simulink model "MySimplifiedTestingModel_2"  (R2023a)
settings: Solver=ode1  StartTime=0.0  StopTime=inf  FixedStep=0.001  RelTol=1e-3
PostLoadFcn:
  | , if any(exist('dsrtsu_mdlpostloadfcn', 'file') ~= 0), dsrtsu_mdlpostloadfcn('Execute', bdroot); end,
InitFcn:
  | , if any(exist('rtifpga_mdlclblib', 'file') ~= 0), rtifpga_mdlclblib('Init', bdroot); end,
model workspace (MAT data in the model file):
  mode = 2
libraries: rti1202serlib x5, simulink x2
(part 1 of 2)
Description:
  | Standard RTI1202 template.
  | Supported MATLAB version:  R2023a.
settings Model: Tag=RTI1202  DSRTSU_INTERNAL_RTI_VER=620  DSRTSU_INTERNAL_RTI_TYPE=rti1202  RTICANMMDATA=struct('GeneralSetupData',struct('modelroot','C:\Users\VM-User\Desktop\MigrationScripts','generalsettings',struct('filesettings',struct('destfolder',struct('Name','RTICANMM_FILES','Check',1),'buildfolder',struct('Name','.','Check',1),'AbsDestfolder',struct('Name','C:\Users\VM-User\Desktop\MigrationScripts\RTICANMM_FILES'),'AbsBuildfolder',struct('Name','C:\Users\VM-User\Desktop\MigrationScripts'))),'options',struct('addpaths',1,'rmpaths',1,'addtrcexclusion',true,'cannavigator',struct('checkmonitoring',0),'show_usrtrc',0,'use_usrtrc',0),'advanced',struct('options',ones(1,100)),'MPSetup',{{}},'RTI',struct('Type','RTI1202','Ver','7.17','Date','02-Nov-2021'),'modelname','','block','untitled'))  DSRTSU_INTERNAL_RTIFPGA=200  DSRTSU_INTERNAL_RTISTBM_VER=23.1  Creator=yd12yqyf  LastModifiedBy=ej62ixyv
settings SolverCC: AlgebraicLoopSolver=TrustRegion
settings DataIOCC: ReturnWorkspaceOutputs=off
settings OptimizationCC: BlockReduction=off  OptimizeBlockIOStorage=off  BufferReuse=off  ReuseModelBlockBuffer=off  GlobalBufferReuse=off  ExpressionFolding=off  LocalBlockOutputs=off  OptimizeDataStoreBuffers=off  BusAssignmentInplaceUpdate=off
settings DebuggingCC: UnderSpecifiedDataTypeMsg=warning  UnconnectedInputMsg=warning  UnconnectedOutputMsg=warning  UnconnectedLineMsg=warning  PregeneratedLibrarySubsystemCodeDiagnostic=none  UnderSpecifiedDimensionMsg=warning  ArithmeticOperatorsInVariantConditions=warning
settings HardwareCC: ProdBitPerPointer=32  ProdBitPerSizeT=32  ProdBitPerPtrDiffT=32  ProdLargestAtomicInteger=Integer  ProdEndianess=BigEndian  ProdWordSize=32  ProdLongLongMode=on  ProdHWDeviceType=Custom Processor->Custom  TargetIntDivRoundTo=Zero  TargetEndianess=BigEndian  TargetHWDeviceType=Custom Processor->Custom
settings ModelReferenceCC: EnableRefExpFcnMdlSchedulingChecks=on  EnableParallelModelReferenceBuilds=on  ParallelModelReferenceMATLABWorkerInit=Load Top Model
settings SFSimCC: SimUseLocalCustomCode=off  MATLABDynamicMemAlloc=off  CustomCodeUndefinedFunction=UseInterfaceOnly
settings RTWCC: Description=dSPACE DS1202 Hardware Platform  SystemTargetFile=rti1202.tlc  MakeCommand=make_rti  TemplateMakefile=rti1202.tmf  RTWUseLocalCustomCode=off  DLArmComputeVersion=19.05
settings CodeAppCC: StateflowObjectComments=on
settings STFCustomTargetCC: ParMdlRefBuildCompliant=on  ConcurrentExecutionCompliant=off  GRTInterface=off  UseToolchainInfoCompliant=off  SystemTargetFile=rti1202.tlc
settings GRTTargetCC: CompOptLevelCompliant=off  ConcurrentExecutionCompliant=off  CombineOutputUpdateFcns=off  MatFileLogging=off  CPPClassGenCompliant=off  UseToolchainInfoCompliant=off
settings ConfigComp: CovMetricSettings=dswe

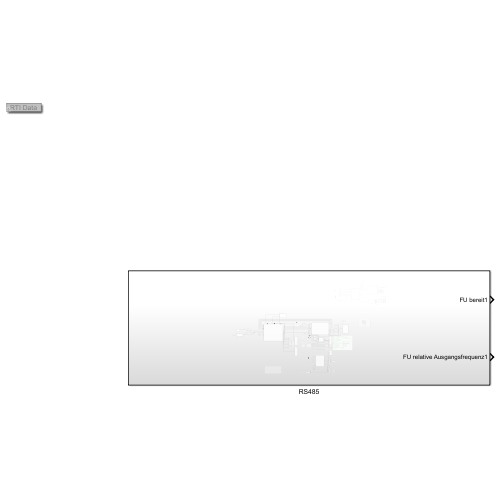
[thumbnail: Simulink's stored preview of the top-level diagram]
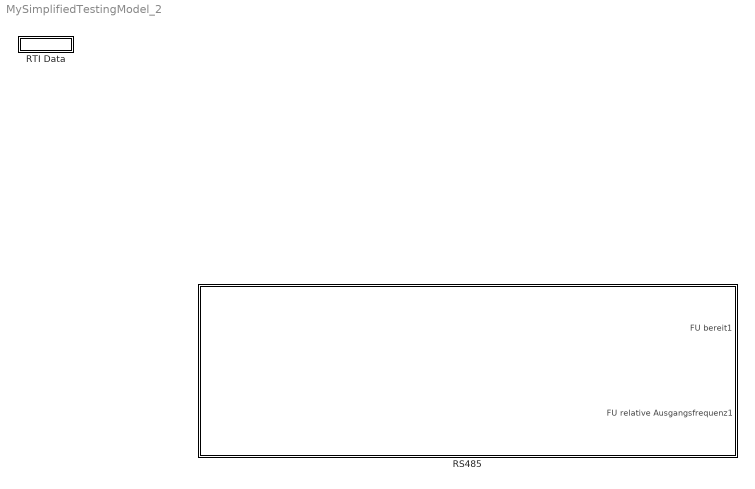
== system MySimplifiedTestingModel_2 ==
  RS485 : Subsystem
  RTI Data : Subsystem  Tag=struct('RTIDataServer',struct('RTIDataServerVs','2','RTIModelDescription','struct(''main'',''MySimplifiedTestingModel_2'',''sub'','''',''isMp'',0)'))  LoadFcn="if exist('rtidc'), try,  rtidc('DataHostBlockClbLoad', gcbh); catch, disp(['Warning: ''LoadFcn'' for RTI Data block failed: ' lasterr]); end, end,"  mask(RTI_DATA_HOST){}
      mask help:
      | RTI Data Block.
      | This block is used by RTI to store internal model-dependent data.
      | Please keep this block on the root level of the model. Deleting this block will result in data loss.
      |
      | NEVER DELETE OR COPY THIS BLOCK!
      settings: CopyFcn="if exist('rtidc'), try,  rtidc('DataHostBlockClbCopy', gcbh); catch, disp(['Warning: ''CopyFcn'' for RTI Data block failed: ' lasterr]); end, end,"  DeleteFcn="if exist('rtidc'), try,  rtidc('DataHostBlockClbDelete', gcbh); catch, disp(['Warning: ''DeleteFcn'' for RTI Data block failed: ' lasterr]); end, end,"  ModelCloseFcn="if exist('rtidc'), try,  rtidc('DataHostBlockClbModelClose', gcbh); catch, disp(['Warning: ''ModelCloseFcn'' for RTI Data block failed: ' lasterr]); end, end,"  PreSaveFcn="if exist('rtidc'), try,  rtidc('DataHostBlockClbPreSave', gcbh); catch, disp(['Warning: ''PreSaveFcn'' for RTI Data block failed: ' lasterr]); end, end,"  PostSaveFcn="if exist('rtidc'), try,  rtidc('DataHostBlockClbPostSave', gcbh); catch, disp(['Warning: ''PostSaveFcn'' for RTI Data block failed: ' lasterr]); end, end,"  NameChangeFcn="if exist('rtidc'), try,  rtidc('DataHostBlockClbNameChange', gcbh); catch, disp(['Warning: ''NameChangeFcn'' for RTI Data block failed: ' lasterr]); end, end,"
      mask Help:
      | RTI Data Block.
      | This block is used by RTI to store internal model-dependent data.
      | Please keep this block on the root level of the model. Deleting this block will result in data loss.
      | 
      | NEVER DELETE OR COPY THIS BLOCK!
      mask Display:
      | text(0.5, 0.5, 'RTI Data', 'HorizontalAlignment', 'center');
      | plot([1 0]);

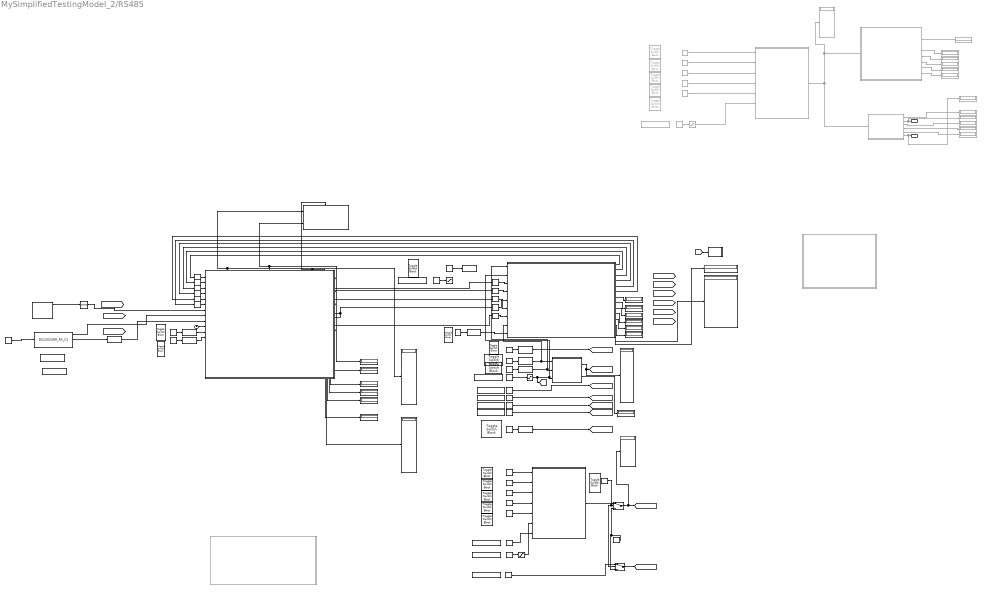
== system MySimplifiedTestingModel_2/RS485 ==
  note: RX_Data
  note: RX_Len
  note: THRE
  note: %| Bit| Bit value = 0 | Bit value = 1 |
      | %|----|--------------------------------------|------------------------------------|
      | %| 00 | selection between the four "3-10 Preset reference [0]...[3]" |
      | %| 01 | --""-- |
      | %|----|--------------------------------------|------------------------------------|
      | %| 02 | DC brake and stop | performs ramp |
      | %|----|--------------------------------------|------------------------------------|
      | %| 03 | lets the motor coast | starts the motor if conditions are met |
      | %|----|--------------------------------------|------------------------------------|
      | %| 04 | motor speed decreases until stop | |
      | %|----|--------------------------------------|------------------------------------|
      | %| 05 | current output frequency is stored | |
      | %|----|--------------------------------------|------------------------------------|
      | %| 06 | stop using ramp time | starts the motor if conditions are met |
      | %|----|--------------------------------------|------------------------------------|
      | %| 07 | no reset | reset |
      | %|----|--------------------------------------|------------------------------------|
      | %| 08 | | output frequency "3-19 Jog [RPM]" |
      | %|----|--------------------------------------|------------------------------------|
      | %| 09 | ramp 1 active ("3-41" and "3-42") | ramp 2 active ("3-51" and "3-52") |
      | %|----|--------------------------------------|------------------------------------|
      | %| 10 | control word is ignored | control word is used |
      | %|----|--------------------------------------|------------------------------------|
      | %| 11 | relay 01 not activated | relay 01 activated |
      | %|----|--------------------------------------|------------------------------------|
      | %| 12 | relay 04 not activated | relay 04 activated |
      | %|----|--------------------------------------|------------------------------------|
      | %| 13 | parameter set selection "0-10" and "8-55" |
      | %| 14 | |
      | %|----|--------------------------------------|------------------------------------|
      | %| 15 | no reversal | reversal |
  note: expect_len_ZKDM
  note: expect_crc_kind_ZKDM
  note: expect_addr_ZKDM
  note: req_len
  note: req_bytes
  note: req_valid
  note: resp_len
  note: resp_data
  note: resp_err_ZKDM
  note: resp_ok_ZKDM
  note: grant_ZKDM
  note: tx data
  note: tx len
  note: tx trigger
  Active : Constant  Value=0
  BUS MASTER FSM : Stateflow chart  TreatAsAtomicUnit=on
      settings: PortSchema="{\"entries\":[{\"content\":{\"sides\":[{\"content\":{\"connectorIds\":[\"In4\",\"In16\",\"In18\",\"In8\",\"In14\",\"In10\",\"In1\",\"In2\",\"In3\",\"In6\",\"In11\",\"In12\",\"In5\",\"In15\",\"In17\",\"In7\",\"In13\",\"In9\"]},\"type\":\"ConnectorPlacement.EquallySpacedRectSide\",\"uuid\":\"833d115e-8081-4cb1-98c4-083d374565ad\"},{\"content\":{\"connectorIds\":[\"Out4\",\"Out6\",\"Out5\",\"Out7\",\"Out9\",\"Out10\",\"Out11\",\"Out8\"],\"side\":\"RIGHT\"},\"type\":\"ConnectorPlacement.EquallySpacedRectSide\",\"uuid\":\"f0cbf871-5cea-4f22-8059-874c69130aa3\"},{\"content\":{\"connectorIds\":[\"Out1\",\"Out2\",\"Out3\"],\"side\":\"TOP\"},\"type\":\"ConnectorPlacement.EquallySpacedRectSide\",\"uuid\":\"9def79f2-ef8f-4b80-a903-98ac734b5ab3\"}]},\"type\":\"ConnectorPlacement.EquallySpacedConnector\",\"uuid\":\"db046b19-190e-410f-b654-5051c870f3be\"}],\"packageUris\":[\"http://schema.mathworks.com/mf0/Connector/R2020b\"],\"version\":\"1.0\"}"
  Begrenzung Arbeitstemperatur1 : Saturate  UpperLimit=100  LowerLimit=0  OutDataTypeStr=uint8
  Begrenzung Arbeitstemperatur2 : Saturate  Commented=on  UpperLimit=100  LowerLimit=0
  Begrenzung Arbeitstemperatur3 : Saturate  UpperLimit=100  LowerLimit=0
  Bit Index 6: Transmitter holding register empty (THRE) indicator1 : Selector  InputPortWidth=8  IndexOptions=Starting index (dialog)  Indices=[6]  OutputSizes=1
  Cast : DataTypeConversion  OutDataTypeStr=uint8  SaturateOnIntegerOverflow=off  RndMeth=Floor
  Cast To Boolean{,1..7} (8 alike) : DataTypeConversion  OutDataTypeStr=boolean  SaturateOnIntegerOverflow=off  RndMeth=Floor
  Clock : Clock
  Constant1 : Constant
  Constant10 : Constant
  Constant11 : Constant  Value=34
  Constant12 : Constant  Value=8  OutDataTypeStr=uint8
  Constant13 : Constant  Value=125
  Constant14 : Constant  Value=0
  Constant15 : Constant  Value=0  OutDataTypeStr=uint8
  Constant16 : Constant  Value=0
  Constant19 : Constant  Value=8  OutDataTypeStr=uint32
  Constant2 : Constant  Commented=on  Value=34
  Constant5 : Constant  Value=0
  Constant6 : Constant  Value=12  OutDataTypeStr=uint8
  Constant7 : Constant  Value=31  OutDataTypeStr=uint8
  Constant8 : Constant  Value=8  OutDataTypeStr=uint8
  ConstantSwitch{1,3..6} (5 alike) : Constant  Commented=on
  ConstantSwitch{2,8..11} (5 alike) : Constant  Value=0
  ConstantSwitch7 : Constant
  Create 8-Bytes Command : MATLAB Function  TreatAsAtomicUnit=on
  DS1202SER_RX_C2 : rti1202serlib/DS1202SER_RX_C1  Reserved1=[]  Reserved2=[]  Reserved3=[]  Reserved4=[]  DSProperties=struct('RTI',struct('IOBoardType',{{'DS1202','SER'}},'SlaveProcessor','NONE','Version',uint32(1),'BlockType',struct('isSLSource',uint8(1),'isSLSink',uint8(1),'isHWSource',uint8(0),'isHWSink',uint8(1),'isSetup',uint8(0),'isInline',uint8(1),'isNonInline',uint8(0),'isInterrupt',uint8(0),'isChannelwise',uint8(1)),'UnitType','GENSER','Identifier','RECEIVE','DialogType','ML','BlockSet','NONE'))  RTIBlockInterface=struct('BlockName',struct('Token',{{'DS1202SER_RX_C'}},'BlockParam',{{'ChannelNo'}}),'InputPortsWidth',int32(1),'InputPortsActive',1,'InputPortsDataType',{{'SS_UINT32'}},'InputPortsName',{{'NumBytes'}},'OutputPortsWidth',int32([127 1 1]),'OutputPortsActive',[1 1 1],'OutputPortsDataType',{{'SS_UINT8','SS_UINT32','SS_INT32'}},'OutputPortsName',{{'RXBytes','NumRXBytes','Status'}},'BlockDisplay',{{['Serial Receive'],'center'}},'IconTransparency','on','ParameterTunableNames',{{'BytesRefNumOf'}},'InitLevel',2,'DialogFcn','guigenserreceive','MaskDescription',['To read data from the UART SW FIFO.'])  RTIBlockParameters=struct('BoardNo',{{1,'ON',[1 1]}},'ChannelNo',{{2,'ON',[1 2]}},'ChannelNumOf',{{2,'OFF',[]}},'ReceptionDataMode',{{2,'OFF',[]}},'ParamTunableMode',{{1,'OFF',[]}},'BytesRefNumOfT',{{'1','OFF',[1 inf]}},'BytesRefNumOfNT',{{'1','OFF',[1 inf]}},'BytesRefNumOfMax',{{'127','OFF',[1 inf]}},'BytesRefNumOfMode',{{0,'OFF',[]}},'BytesActNumOfMode',{{1,'OFF',[]}},'ReceptionStatusMode',{{1,'OFF',[]}},'FifoSizeDefault',{{64,'OFF',[]}},'TLCFileName',{{'rtigenserreceive','OFF',[]}})  RTISFcnParameters=struct('BoardNo','double','ChannelNo','double','ChannelNumOf','double','ReceptionDataMode','double','ParamTunableMode','double','BytesRefNumOfT','double','BytesRefNumOfNT','double','BytesRefNumOfMax','double','BytesRefNumOfMode','double','BytesActNumOfMode','double','ReceptionStatusMode','double','TLCFileName','char')  RTIBlockParaDefault=struct('BoardNo',1,'ChannelNo',1,'ChannelNumOf',2,'ReceptionDataMode',1,'ParamTunableMode',1,'BytesRefNumOfT',1,'BytesRefNumOfNT',1,'BytesRefNumOfMax',1,'BytesRefNumOfMode',0,'BytesActNumOfMode',1,'ReceptionStatusMode',1,'FifoSizeDefault',64,'TLCFileName','rtigenserreceive')
  DS1202SER_SETUP_C1 : rti1202serlib/DS1202SER_SETUP_C1  Reserved1=[]  Reserved2=[]  Reserved3=[]  Reserved4=[]  DSProperties=struct('RTI',struct('Version',uint32(2),'IOBoardType',{{'DS1202','SER'}},'SlaveProcessor','NONE','BlockType',struct('isSLSource',uint8(0),'isSLSink',uint8(0),'isHWSource',uint8(0),'isHWSink',uint8(0),'isSetup',uint8(1),'isInline',uint8(1),'isNonInline',uint8(0),'isInterrupt',uint8(0),'isChannelwise',uint8(1)),'UnitType','GENSER','Identifier','SETUP','DialogType','ML','BlockSet','NONE'))  RTIBlockInterface=struct('BlockName',struct('Token',{{'DS1202SER_SETUP_C'}},'BlockParam',{{'ChannelNo'}}),'BlockDisplay',{{['Serial Setup'],'center'}},'IconTransparency','off','ParameterTunableNames',{{}},'InitLevel',1,'DialogFcn','guigensersetup','MaskDescription',['To set the global specifications for the UART interface.'])  RTIBlockParameters=struct('ParityMode',{{3,'OFF',[1 5]}},'TransceiverMode',{{[3;1],'OFF',[]}},'QuartzFrequency',{{'160000000','OFF',[]}},'BoardNo',{{1,'ON',[1 1]}},'ChannelNo',{{1,'ON',[1 2]}},'ChannelNumOf',{{2,'OFF',[]}},'BaudRate',{{'9600','OFF',[]}},'DataBitsNumOf',{{4,'OFF',[1 4]}},'StopBitsNumOf',{{1,'OFF',[1 3]}},'ReceiveIntLevelUart',{{1,'OFF',[1 4]}},'AutoflowMode',{{0,'OFF',[]}},'FifoSize',{{'128','OFF',[]}},'ReceiveIntLevelFifo',{{0,'OFF',[]}},'FifoOverrunMode',{{1,'OFF',[]}},'FifoBlockSize',{{'0','OFF',[]}},'TermMode',{{1,'OFF',[]}},'TLCFileName',{{'rtigensersetup','OFF',[]}})  RTISFcnParameters=struct('BoardNo','double','ChannelNo','double','ChannelNumOf','double','BaudRate','double','DataBitsNumOf','double','StopBitsNumOf','double','ParityMode','double','TransceiverMode','double','ReceiveIntLevelUart','double','AutoflowMode','double','FifoSize','double','ReceiveIntLevelFifo','double','FifoBlockSize','double','TermMode','double','QuartzFrequency','double','TLCFileName','char')  RTIBlockParaDefault=struct('ParityMode',1,'TransceiverMode',[1;1],'QuartzFrequency',160000000,'BoardNo',1,'ChannelNo',1,'ChannelNumOf',2,'BaudRate',115200,'DataBitsNumOf',4,'StopBitsNumOf',1,'ReceiveIntLevelUart',4,'AutoflowMode',0,'FifoSize',64,'ReceiveIntLevelFifo',0,'FifoOverrunMode',1,'FifoBlockSize',0,'TermMode',1,'TLCFileName','rtigensersetup')
  DS1202SER_SETUP_C2 : rti1202serlib/DS1202SER_SETUP_C1  Reserved1=[]  Reserved2=[]  Reserved3=[]  Reserved4=[]  DSProperties=struct('RTI',struct('Version',uint32(2),'IOBoardType',{{'DS1202','SER'}},'SlaveProcessor','NONE','BlockType',struct('isSLSource',uint8(0),'isSLSink',uint8(0),'isHWSource',uint8(0),'isHWSink',uint8(0),'isSetup',uint8(1),'isInline',uint8(1),'isNonInline',uint8(0),'isInterrupt',uint8(0),'isChannelwise',uint8(1)),'UnitType','GENSER','Identifier','SETUP','DialogType','ML','BlockSet','NONE'))  RTIBlockInterface=struct('BlockName',struct('Token',{{'DS1202SER_SETUP_C'}},'BlockParam',{{'ChannelNo'}}),'BlockDisplay',{{['Serial Setup'],'center'}},'IconTransparency','off','ParameterTunableNames',{{}},'InitLevel',1,'DialogFcn','guigensersetup','MaskDescription',['To set the global specifications for the UART interface.'])  RTIBlockParameters=struct('ParityMode',{{3,'OFF',[1 5]}},'TransceiverMode',{{[3;3],'OFF',[]}},'QuartzFrequency',{{'160000000','OFF',[]}},'BoardNo',{{1,'ON',[1 1]}},'ChannelNo',{{2,'ON',[1 2]}},'ChannelNumOf',{{2,'OFF',[]}},'BaudRate',{{'9600','OFF',[]}},'DataBitsNumOf',{{3,'OFF',[1 4]}},'StopBitsNumOf',{{1,'OFF',[1 3]}},'ReceiveIntLevelUart',{{1,'OFF',[1 4]}},'AutoflowMode',{{0,'OFF',[]}},'FifoSize',{{'128','OFF',[]}},'ReceiveIntLevelFifo',{{0,'OFF',[]}},'FifoOverrunMode',{{1,'OFF',[]}},'FifoBlockSize',{{'0','OFF',[]}},'TermMode',{{1,'OFF',[]}},'TLCFileName',{{'rtigensersetup','OFF',[]}})  RTISFcnParameters=struct('BoardNo','double','ChannelNo','double','ChannelNumOf','double','BaudRate','double','DataBitsNumOf','double','StopBitsNumOf','double','ParityMode','double','TransceiverMode','double','ReceiveIntLevelUart','double','AutoflowMode','double','FifoSize','double','ReceiveIntLevelFifo','double','FifoBlockSize','double','TermMode','double','QuartzFrequency','double','TLCFileName','char')  RTIBlockParaDefault=struct('ParityMode',1,'TransceiverMode',[1;1],'QuartzFrequency',160000000,'BoardNo',1,'ChannelNo',1,'ChannelNumOf',2,'BaudRate',115200,'DataBitsNumOf',4,'StopBitsNumOf',1,'ReceiveIntLevelUart',4,'AutoflowMode',0,'FifoSize',64,'ReceiveIntLevelFifo',0,'FifoOverrunMode',1,'FifoBlockSize',0,'TermMode',1,'TLCFileName','rtigensersetup')
  DS1202SER_STAT_C1 : rti1202serlib/DS1202SER_STAT_C1  Reserved1=[]  Reserved2=[]  Reserved3=[]  Reserved4=[]  DSProperties=struct('RTI',struct('IOBoardType',{{'DS1202','SER'}},'SlaveProcessor','NONE','Version',uint32(1),'BlockType',struct('isSLSource',uint8(1),'isSLSink',uint8(0),'isHWSource',uint8(0),'isHWSink',uint8(0),'isSetup',uint8(0),'isInline',uint8(1),'isNonInline',uint8(0),'isInterrupt',uint8(0),'isChannelwise',uint8(1)),'UnitType','GENSER','Identifier','STATUS','DialogType','ML','BlockSet','NONE'))  RTIBlockInterface=struct('BlockName',struct('Token',{{'DS1202SER_STAT_C'}},'BlockParam',{{'ChannelNo'}}),'OutputPortsWidth',int32([8 8 8]),'OutputPortsActive',[1 1 1],'OutputPortsName',{{'Line','Modem','Interrupt'}},'OutputPortsDataType',{{'SS_BOOLEAN','SS_BOOLEAN','SS_BOOLEAN'}},'BlockDisplay',{{['Serial Status'],'left'}},'IconTransparency','on','ParameterTunableNames',{{}},'InitLevel',1,'DialogFcn','guigenserstatus','MaskDescription',['To read the contents of the UART status register.'])  RTIBlockParameters=struct('BoardNo',{{1,'ON',[1 1]}},'ChannelNo',{{1,'ON',[1 2]}},'ChannelNumOf',{{2,'OFF',[]}},'LineStatUartMode',{{1,'OFF',[]}},'ModemStatUartMode',{{1,'OFF',[]}},'InterruptStatUartMode',{{1,'OFF',[]}},'TLCFileName',{{'rtigenserstatus','OFF',[]}})  RTISFcnParameters=struct('BoardNo','double','ChannelNo','double','ChannelNumOf','double','LineStatUartMode','double','ModemStatUartMode','double','InterruptStatUartMode','double','TLCFileName','char')  RTIBlockParaDefault=struct('BoardNo',1,'ChannelNo',1,'ChannelNumOf',2,'LineStatUartMode',1,'ModemStatUartMode',1,'InterruptStatUartMode',1,'TLCFileName','rtigenserstatus')
  Display{,1,9,16..31} (19 alike) : Display
      Display19 settings: Decimation=16
      Display21 settings: Decimation=16
      Display22 settings: Decimation=16
      Display25 settings: Decimation=8
      Display30 settings: Format=binary (Stored Integer)  Decimation=8
      Display31 settings: Format=binary (Stored Integer)
  Display{2..8,10..15} (13 alike) : Display  Commented=on
      Display15 settings: Decimation=8
  Edit{,3..10} (9 alike) : EditField  LabelPosition=Hide  ShowInitialText=on  Alignment=Center
  Edit2 : EditField  Commented=on  LabelPosition=Hide  ShowInitialText=on  Alignment=Center
  From : From
  Goto : Goto
  Invalid CTW : Constant  Value=0
  Length : Constant  Value=6  OutDataTypeStr=uint8
  MATLAB Function : MATLAB Function  TreatAsAtomicUnit=on
  MATLAB Function2 : MATLAB Function  Commented=on  TreatAsAtomicUnit=on
  MATLAB Function3 : MATLAB Function  Commented=on  TreatAsAtomicUnit=on
  MATLAB Function4 : MATLAB Function  TreatAsAtomicUnit=on
  Memory{,1..10} (11 alike) : Memory
  RX on : Constant  Value=0
  Saturation : Saturate  UpperLimit=100  LowerLimit=0
  Setpoint : Constant  Value=100
  Subsystem : Subsystem
  Subsystem2 : Subsystem  Commented=on
  Switch : Switch  Criteria=u2 > Threshold  SaturateOnIntegerOverflow=off  InputSameDT=off
  Switch1 : Switch  Criteria=u2 > Threshold  SaturateOnIntegerOverflow=off  InputSameDT=off
  THERMO FSM : Stateflow chart  Commented=on  TreatAsAtomicUnit=on
  TX on : Constant
  Toggle Switch{2,8..20} (14 alike) : ToggleSwitchBlock
      settings: Values={{'Off', 'On'}, [0 1]}
  Toggle Switch{3..7} (5 alike) : ToggleSwitchBlock  Commented=on
      settings: Values={{'Off', 'On'}, [0 1]}
  Variant Subsystem : Subsystem  Commented=on  Variant=on
  ZKDM FSM : Stateflow chart  TreatAsAtomicUnit=on
  FU bereit1 : Outport
  FU relative Ausgangsfrequenz1 : Outport  Port=2
  wires:
  Constant1/1 -> Begrenzung Arbeitstemperatur1/1
  Clock/1 -> BUS MASTER FSM/6(now)
  BUS MASTER FSM/4(grant_ZKDM) -> Memory/1, Display16/1
  BUS MASTER FSM/6(resp_ok_ZKDM) -> Memory1/1, Display17/1
  BUS MASTER FSM/5(resp_err_ZKDM) -> Memory2/1, Display18/1
  BUS MASTER FSM/7(resp_data) -> Display19/1, Memory3/1
  BUS MASTER FSM/9(resp_len) -> Memory4/1, Display20/1
  BUS MASTER FSM/1(TX_Data) -> Subsystem/1(TXBytes), Display22/1
  BUS MASTER FSM/2(TX_Len) -> Subsystem/2(NumBytes), Display23/1
  BUS MASTER FSM/3(TX_Trigger) -> Subsystem/Trigger, Display24/1
  ZKDM FSM/1(req_valid) -> Memory5/1
  ZKDM FSM/2(req_bytes) -> Memory6/1
  ZKDM FSM/3(req_len) -> Memory7/1
  ZKDM FSM/4(expect_addr_ZKDM) -> Memory8/1
  ZKDM FSM/6(expect_len_ZKDM) -> Memory9/1
  ZKDM FSM/5(expect_crc_kind_ZKDM) -> Memory10/1
  MATLAB Function3/1(u) -> Subsystem2/1(Antworttelegramm), Display15/1, MATLAB Function2/1(u)
  Begrenzung Arbeitstemperatur2/1 -> MATLAB Function3/6(freq_rel_percent)
  Constant2/1 -> Begrenzung Arbeitstemperatur2/1
  ConstantSwitch1/1 -> MATLAB Function3/1(fu_ctrl_ready)
  ConstantSwitch3/1 -> MATLAB Function3/2(fu_ready)
  ConstantSwitch4/1 -> MATLAB Function3/3(fault_trip)
  ConstantSwitch5/1 -> MATLAB Function3/4(fault_no_trip)
  ConstantSwitch6/1 -> MATLAB Function3/5(bus_control_active)
  MATLAB Function2/3(freq_rel_percent) -> Display2/1
  MATLAB Function2/5(fu_ctrl_ready) -> Display3/1
  MATLAB Function2/6(fu_ready) -> Display4/1
  MATLAB Function2/7(fault_trip) -> Display5/1
  MATLAB Function2/8(fault_no_trip) -> Display6/1
  MATLAB Function2/9(bus_control_active) -> Display7/1
  Subsystem2/5(Bussteuerung aktive) -> Display14/1
  Subsystem2/2(FU bereit) -> Display11/1, FU bereit1/1
  Subsystem2/1(Steuerung FU bereit) -> Display10/1
  Subsystem2/6(relative Ausgangsfrequenz) -> Display8/1, FU relative Ausgangsfrequenz1/1
  Subsystem2/3(Fehler mit Abschaltung) -> Display12/1
  Subsystem2/4(Fehler ohne Abschaltung) -> Display13/1
  Cast To Boolean/1 -> ZKDM FSM/8(invalid_flag), Create 8-Bytes Command/1(invalid_control_word)
  Cast To Boolean1/1 -> ZKDM FSM/1(active), Create 8-Bytes Command/2(active)
  Saturation/1 -> Goto/1, Create 8-Bytes Command/3(setpoint), ZKDM FSM/2(setpoint)
  Invalid CTW/1 -> Cast To Boolean/1
  Active/1 -> Cast To Boolean1/1
  Setpoint/1 -> Saturation/1
  Constant5/1 -> Cast To Boolean2/1
  Constant6/1 -> [expect_addr_ZKDM]
  Constant7/1 -> [expect_crc_kind_ZKDM]
  Constant8/1 -> [expect_len_ZKDM]
  Length/1 -> [req_len]
  Cast To Boolean2/1 -> [req_valid]
  Create 8-Bytes Command/1(command) -> Display21/1, [req_bytes]
  Cast To Boolean3/1 -> [THRE]
  Constant10/1 -> Cast To Boolean3/1
  Begrenzung Arbeitstemperatur3/1 -> MATLAB Function4/6(freq_rel_percent)
  ConstantSwitch10/1 -> MATLAB Function4/4(fault_no_trip)
  ConstantSwitch8/1 -> MATLAB Function4/2(fu_ready)
  ConstantSwitch11/1 -> MATLAB Function4/5(bus_control_active)
  Constant11/1 -> Begrenzung Arbeitstemperatur3/1
  ConstantSwitch7/1 -> MATLAB Function4/1(fu_ctrl_ready)
  MATLAB Function4/1(u) -> Switch/1
  ConstantSwitch9/1 -> MATLAB Function4/3(fault_trip)
  Constant12/1 -> Switch1/1
  Bit Index 6: Transmitter holding register empty (THRE) indicator1/1 -> BUS MASTER FSM/1(THRE)
  DS1202SER_RX_C2/1 -> BUS MASTER FSM/2(RX_Data)
  Constant13/1 -> MATLAB Function4/7(addr)
  Switch/1 -> Display25/1, [RX_Data]
  Constant14/1 -> Switch1/2, Switch/2
  Constant15/1 -> Switch1/3, Switch/3
  Switch1/1 -> [RX_Len]
  ConstantSwitch2/1 -> Cast To Boolean4/1
  Memory1/1 -> ZKDM FSM/4(resp_ok)
  Memory/1 -> ZKDM FSM/3(grant)
  Memory2/1 -> ZKDM FSM/6(resp_err)
  Memory3/1 -> ZKDM FSM/5(resp_data)
  Memory4/1 -> ZKDM FSM/7(resp_len)
  Memory5/1 -> BUS MASTER FSM/4(req_valid_ZKDM)
  Memory6/1 -> BUS MASTER FSM/16(req_bytes_ZKDM)
  Memory7/1 -> BUS MASTER FSM/18(req_len_ZKDM)
  Memory8/1 -> BUS MASTER FSM/8(expect_addr_ZKDM)
  Memory9/1 -> BUS MASTER FSM/14(expect_len_ZKDM)
  Memory10/1 -> BUS MASTER FSM/10(expect_crc_kind_ZKDM)
  Constant16/1 -> Cast To Boolean5/1
  Cast To Boolean5/1 -> ZKDM FSM/9(tx_trigger)
  Cast To Boolean6/1 -> BUS MASTER FSM/11(tx_switch)
  TX on/1 -> Cast To Boolean6/1
  Cast To Boolean7/1 -> BUS MASTER FSM/12(rx_switch)
  DS1202SER_STAT_C1/1 -> Bit Index 6: Transmitter holding register empty (THRE) indicator1/1
  Cast/1 -> BUS MASTER FSM/3(RX_Len)
  Constant19/1 -> DS1202SER_RX_C2/1
  DS1202SER_RX_C2/2 -> Cast/1
  ZKDM FSM/7(fault_no_trip) -> Display/1
  ZKDM FSM/8(fault_trip) -> Display1/1
  ZKDM FSM/9(fu_ctrl_ready) -> Display9/1
  ZKDM FSM/10(fu_ready) -> Display26/1
  ZKDM FSM/11(bus_ctrl_active) -> Display27/1
  ZKDM FSM/12(freq_rel) -> Display28/1
  RX on/1 -> Cast To Boolean7/1
  Create 8-Bytes Command/2(pcd2) -> Display29/1
  ZKDM FSM/13(debug_command) -> Display30/1
  From/1 -> MATLAB Function/1(setpoint)
  ZKDM FSM/14(debug_pcd2) -> Display31/1

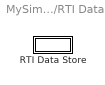
== system MySimplifiedTestingModel_2/RTI Data ==
  RTI Data Store : Subsystem  Tag="struct('private',struct('version',struct('dsVer',uint32(2)),'access',struct('modified',['19-Feb-2026 09:09:14'],'type','Model','isPerm',1)),'public',struct('main',struct('data',[]),'sub',struct('name',{{'MySimplifiedTestingModel_2'}},'data',{{struct('TH',struct('thTaskInfo',struct('taskType',{'TIMER','HWINT','TMRINT','SWINT','GLINT'},'tasksNumOf',{1,0,0,0,0},'srcIds',{{'TIMERA'},{},{},{},{}},'taskNames',{{['Timer Task 1']},{},{},{},{}})),'th_tc',struct('dataType','TASK','taskGroupId','','taskGroupList',{{}},'taskSchedulingPolicy','FCFS','taskType','TIMER','blkh',-1,'srcId','TIMERA','srcSgnName',['Timer A interrupt'],'srcCpuName','','taskName',['Timer Task 1  [0.001] s'],'taskNameDisplayExt','','smplTime',0.001,'smplTimeOffs',0,'hasFixedPriority',0,'priority',1,'hasFixedOvc',0,'ovcType',1,'ovcMax',1),'tc_th',struct('dataType','TASK','taskGroupId','','taskGroupList',{{}},'taskSchedulingPolicy','FCFS','taskType','TIMER','blkh',-1,'srcId','TIMERA','srcSgnName',['Timer A interrupt'],'srcCpuName','','taskName',['Timer Task 1  [0.001] s'],'taskNameDisplayExt','','smplTime',0.001,'smplTimeOffs',0,'hasFixedPriority',0,'priority',1,'hasFixedOvc',0,'ovcType',1,'ovcMax',1))}})))"  mask(RTI_DATA_STORE){}
      mask help:
      | RTI Data Store Block. This block is used by RTI to store internal model dependent data. Deleting this block will result in data loss.
      |
      | NEVER DELETE, COPY, OR MODIFY THIS BLOCK!
      mask Help:
      | RTI Data Store Block. This block is used by RTI to store internal model dependent data. Deleting this block will result in data loss.
      | 
      | NEVER DELETE, COPY, OR MODIFY THIS BLOCK!
      mask Display: text(0.5, 0.5, ' ', 'HorizontalAlignment', 'center');

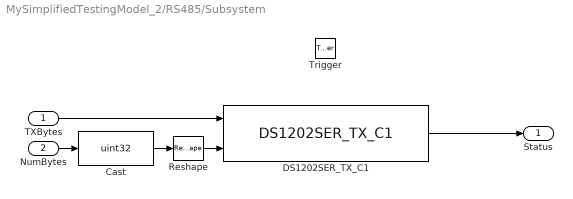
== system MySimplifiedTestingModel_2/RS485/Subsystem ==
  TXBytes : Inport
  NumBytes : Inport  Port=2
  Trigger : TriggerPort  VariantControl=(inherit)  PortDimensions=1
  Cast : DataTypeConversion  OutDataTypeStr=uint32  SaturateOnIntegerOverflow=off  RndMeth=Floor
  DS1202SER_TX_C1 : rti1202serlib/DS1202SER_TX_C1  Reserved1=[]  Reserved2=[]  Reserved3=[]  Reserved4=[]  DSProperties=struct('RTI',struct('IOBoardType',{{'DS1202','SER'}},'SlaveProcessor','NONE','Version',uint32(1),'BlockType',struct('isSLSource',uint8(1),'isSLSink',uint8(1),'isHWSource',uint8(1),'isHWSink',uint8(0),'isSetup',uint8(0),'isInline',uint8(1),'isNonInline',uint8(0),'isInterrupt',uint8(0),'isChannelwise',uint8(1)),'UnitType','GENSER','Identifier','TRANSMIT','DialogType','ML','BlockSet','NONE'))  RTIBlockInterface=struct('BlockName',struct('Token',{{'DS1202SER_TX_C'}},'BlockParam',{{'ChannelNo'}}),'InputPortsWidth',int32([127 1]),'InputPortsActive',[1 1],'InputPortsDataType',{{'SS_UINT8','SS_UINT32'}},'InputPortsName',{{'TXBytes','NumBytes'}},'OutputPortsWidth',int32([1 1]),'OutputPortsActive',[0 1],'OutputPortsDataType',{{'SS_UINT32','SS_INT32'}},'OutputPortsName',{{'NumTXBytes','Status'}},'BlockDisplay',{{['Serial Transmit'],'center'}},'IconTransparency','on','ParameterTunableNames',{{'BytesRefNumOf'}},'InitLevel',2,'DialogFcn','guigensertransmit','MaskDescription',['To write data to the UART SW FIFO.'])  RTIBlockParameters=struct('BoardNo',{{1,'ON',[1 1]}},'ChannelNo',{{1,'ON',[1 2]}},'ChannelNumOf',{{2,'OFF',[]}},'TransmitFifoOverrunMode',{{1,'OFF',[]}},'ParamTunableMode',{{1,'OFF',[]}},'BytesRefNumOfT',{{'32','OFF',[1 inf]}},'BytesRefNumOfNT',{{'64','OFF',[1 inf]}},'BytesRefNumOfMax',{{'127','OFF',[1 inf]}},'BytesRefNumOfMode',{{0,'OFF',[]}},'BytesActNumOfMode',{{0,'OFF',[]}},'TransmissionStatusMode',{{1,'OFF',[]}},'FifoSizeDefault',{{64,'OFF',[]}},'TLCFileName',{{'rtigensertransmit','OFF',[]}})  RTISFcnParameters=struct('BoardNo','double','ChannelNo','double','ChannelNumOf','double','TransmitFifoOverrunMode','double','ParamTunableMode','double','BytesRefNumOfT','double','BytesRefNumOfNT','double','BytesRefNumOfMax','double','BytesRefNumOfMode','double','BytesActNumOfMode','double','TransmissionStatusMode','double','TLCFileName','char')  RTIBlockParaDefault=struct('BoardNo',1,'ChannelNo',1,'ChannelNumOf',2,'TransmitFifoOverrunMode',1,'ParamTunableMode',1,'BytesRefNumOfT',1,'BytesRefNumOfNT',1,'BytesRefNumOfMax',1,'BytesRefNumOfMode',0,'BytesActNumOfMode',1,'TransmissionStatusMode',1,'FifoSizeDefault',64,'TLCFileName','rtigensertransmit')
  Reshape : Reshape
  Status : Outport
  wires:
  TXBytes/1 -> DS1202SER_TX_C1/1
  DS1202SER_TX_C1/1 -> Status/1
  NumBytes/1 -> Cast/1
  Cast/1 -> Reshape/1
  Reshape/1 -> DS1202SER_TX_C1/2

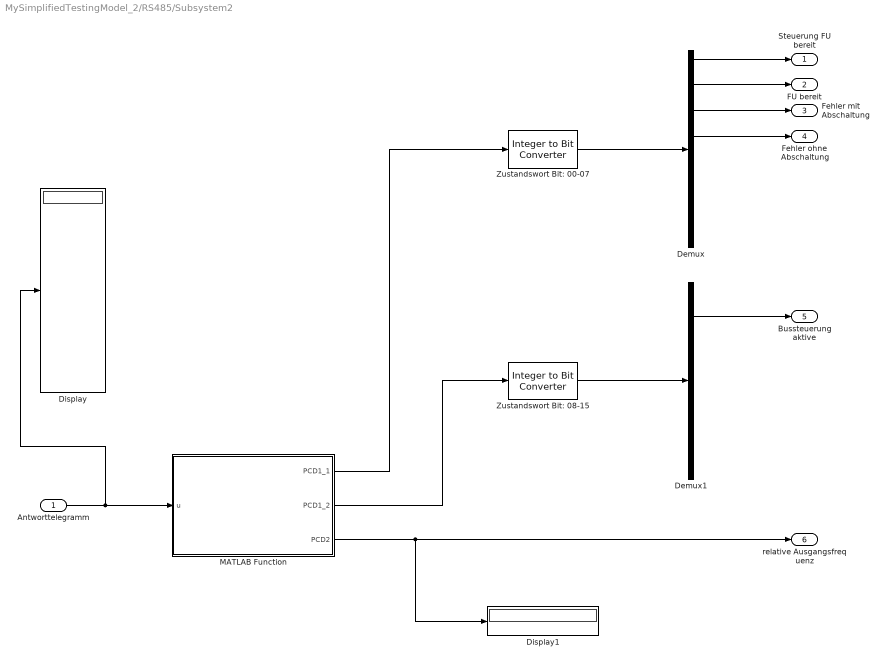
== system MySimplifiedTestingModel_2/RS485/Subsystem2 ==
  Antworttelegramm : Inport
  Demux : Demux  Outputs=8
  Demux1 : Demux  Outputs=8
  Display : Display
      settings: Decimation=8
  Display1 : Display
  MATLAB Function : MATLAB Function  TreatAsAtomicUnit=on
  Zustandswort Bit: 00-07 : simulink/Logic and Bit Operations/Integer to Bit Converter  nbits=8  signedInputValues=Unsigned  bitOrder=MSB first  outDtype=boolean
  Zustandswort Bit: 08-15 : simulink/Logic and Bit Operations/Integer to Bit Converter  nbits=8  signedInputValues=Unsigned  bitOrder=MSB first  outDtype=boolean
  Steuerung FU bereit : Outport
  FU bereit : Outport  Port=2
  Fehler mit Abschaltung : Outport  Port=3
  Fehler ohne Abschaltung : Outport  Port=4
  Bussteuerung aktive : Outport  Port=5
  relative Ausgangsfrequenz : Outport  Port=6
  wires:
  MATLAB Function/3(PCD2) -> Display1/1, relative Ausgangsfrequenz/1
  MATLAB Function/2(PCD1_2) -> Zustandswort Bit: 08-15/1
  MATLAB Function/1(PCD1_1) -> Zustandswort Bit: 00-07/1
  Demux1/2 -> Bussteuerung aktive/1
  Zustandswort Bit: 08-15/1 -> Demux1/1
  Zustandswort Bit: 00-07/1 -> Demux/1
  Demux/4 -> Fehler ohne Abschaltung/1
  Demux/3 -> Fehler mit Abschaltung/1
  Demux/2 -> FU bereit/1
  Demux/1 -> Steuerung FU bereit/1
  Antworttelegramm/1 -> Display/1, MATLAB Function/1(u)

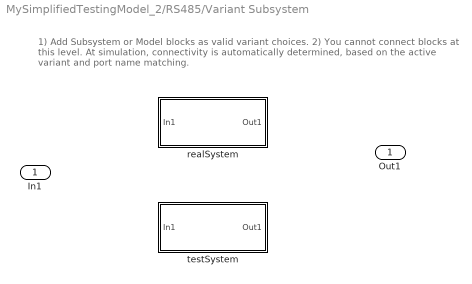
== system MySimplifiedTestingModel_2/RS485/Variant Subsystem ==
  note: 1) Add Subsystem or Model blocks as valid variant choices.
      | 2) You cannot connect blocks at this level. At simulation, connectivity is automatically
      | determined, based on the active variant and port name matching.
  In1 : Inport
  realSystem : Subsystem  VariantControl=mode == 1
  testSystem : Subsystem  VariantControl=mode == 2
  Out1 : Outport

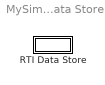
== system MySimplifiedTestingModel_2/RTI Data/RTI Data Store ==
  RTI Data Store : Subsystem  mask(RTI_DATA_STORE){}
      mask help:
      | RTI Data Store Block. This block is used by RTI to store internal model dependent data. Deleting this block will result in data loss.
      |
      | NEVER DELETE, COPY, OR MODIFY THIS BLOCK!
      mask Help:
      | RTI Data Store Block. This block is used by RTI to store internal model dependent data. Deleting this block will result in data loss.
      | 
      | NEVER DELETE, COPY, OR MODIFY THIS BLOCK!
      mask Display: text(0.5, 0.5, ' ', 'HorizontalAlignment', 'center');

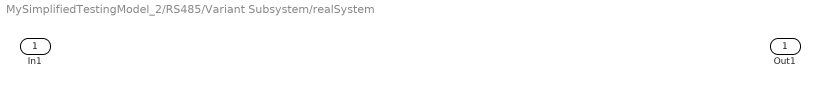
== system MySimplifiedTestingModel_2/RS485/Variant Subsystem/realSystem ==
  In1 : Inport
  Out1 : Outport

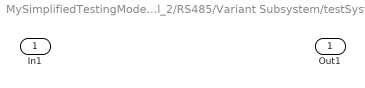
== system MySimplifiedTestingModel_2/RS485/Variant Subsystem/testSystem ==
  In1 : Inport
  Out1 : Outport

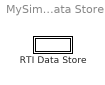
== system MySimplifiedTestingModel_2/RTI Data/RTI Data Store/RTI Data Store ==
  RTI Data Store : Subsystem  mask(RTI_DATA_STORE){}
      mask help:
      | RTI Data Store Block. This block is used by RTI to store internal model dependent data. Deleting this block will result in data loss.
      |
      | NEVER DELETE, COPY, OR MODIFY THIS BLOCK!
      mask Help:
      | RTI Data Store Block. This block is used by RTI to store internal model dependent data. Deleting this block will result in data loss.
      | 
      | NEVER DELETE, COPY, OR MODIFY THIS BLOCK!
      mask Display: text(0.5, 0.5, ' ', 'HorizontalAlignment', 'center');

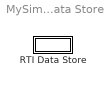
== system MySimplifiedTestingModel_2/RTI Data/RTI Data Store/RTI Data Store/RTI Data Store ==
  RTI Data Store : Subsystem  mask(RTI_DATA_STORE){}
      mask help:
      | RTI Data Store Block. This block is used by RTI to store internal model dependent data. Deleting this block will result in data loss.
      |
      | NEVER DELETE, COPY, OR MODIFY THIS BLOCK!
      mask Help:
      | RTI Data Store Block. This block is used by RTI to store internal model dependent data. Deleting this block will result in data loss.
      | 
      | NEVER DELETE, COPY, OR MODIFY THIS BLOCK!
      mask Display: text(0.5, 0.5, ' ', 'HorizontalAlignment', 'center');

== system MySimplifiedTestingModel_2/RTI Data/RTI Data Store/RTI Data Store/RTI Data Store/RTI Data Store ==

== matlab function MySimplifiedTestingModel_2/RS485/MATLAB Function ==
  data: setpoint input double size=1; y output uint8 size=[1, 2]
function y = fcn(setpoint)
    soll = setpoint * (16384 / 100); 
    pcd2 = typecast(int16(soll),'uint8');
y = pcd2;

== stateflow chart MySimplifiedTestingModel_2/RS485/BUS MASTER FSM ==
  state INIT
    entry:
    TX_Trigger = false;
    TX_Len = 0;
    grant_ZKDM = false;
    grant_THERMO = false;
    resp_ok_ZKDM = false;
    resp_ok_THERMO = false;
    err_ZKDM = uint8(0);
    err_THERMO = uint8(0);
    currentDev = DEV_NONE;
    retry = 0;
    pollCounter = 0;
    rxCount = 0;
  state IDLE
    entry:
    currentDev = DEV_NONE;
    resp_ok_ZKDM=false;
    resp_ok_THERMO=false;
    resp_err_ZKDM=0;
    resp_err_THERMO=0;
    err_ZKDM=0;
    err_THERMO=0;
    grant_ZKDM=false;
    grant_THERMO=false;
    TX_Trigger=false;
    TX_Len=0;
    rxCount=0;
    during:
    if req_valid_ZKDM
    currentDev = DEV_ZKDM;
    elseif (pollCounter >= pollThermoEvery-1) && req_valid_THERMO
    currentDev = DEV_THERMO;
    pollCounter = 0;
    elseif req_valid_THERMO && ~req_valid_ZKDM
    currentDev = DEV_THERMO;
    else
    currentDev = DEV_NONE;
    end
  state VALIDATE1
    (junction 256) -> (junction 196) : {okAddr = addr_ok(rxBuf, rxCount, chosen_expect_addr);
        | okLen  = len_ok(rxCount, chosen_expect_len);
        | okCrc  = crc_ok(rxBuf, rxCount, chosen_expect_crc);}
    (junction 196) -> (junction 197) [order 1] : [~okAddr]
    (junction 196) -> (junction 198) [order 2]
    (junction 197) -> (junction 213)
    (junction 213) -> (junction 214) [order 1] : [currentDev==DEV_ZKDM]
    (junction 213) -> (junction 215) [order 2] : {err_THERMO = ERR_BAD_ADDR;}
    (junction 214) -> (junction 216) : {err_ZKDM = ERR_BAD_ADDR;}
    (junction 216) -> (junction 215)
    (junction 215) -> (junction 205)
    (junction 198) -> (junction 199) [order 1] : [~okLen]
    (junction 198) -> (junction 200) [order 2]
    (junction 199) -> (junction 220)
    (junction 220) -> (junction 221) [order 1] : [currentDev==DEV_ZKDM]
    (junction 220) -> (junction 223) [order 2] : {err_THERMO = ERR_BAD_LEN;}
    (junction 221) -> (junction 227) : {err_ZKDM = ERR_BAD_LEN;}
    (junction 227) -> (junction 223)
    (junction 223) -> (junction 204)
    (junction 200) -> (junction 201) [order 1] : [~okCrc]
    (junction 200) -> (junction 247) [order 2] : {resp_data = rxBuf;
        |     resp_len = rxCount;}
    (junction 201) -> (junction 231)
    (junction 231) -> (junction 232) [order 1] : [currentDev==DEV_ZKDM]
    (junction 231) -> (junction 234) [order 2] : {err_THERMO = ERR_BAD_CRC;}
    (junction 232) -> (junction 238) : {err_ZKDM = ERR_BAD_CRC;}
    (junction 247) -> (junction 248) [order 1] : [currentDev==DEV_ZKDM]
    (junction 238) -> (junction 234)
    (junction 247) -> (junction 249) [order 2] : {resp_ok_THERMO = true;}
    (junction 248) -> (junction 250) : {resp_ok_ZKDM = true;}
    (junction 234) -> (junction 235)
    (junction 250) -> (junction 249)
    (junction 249) -> (junction 202)
    (junction 235) -> (junction 202) [order 2]
    (junction 204) -> (junction 235)
    (junction 205) -> (junction 204)
  state LOAD_REQ
    entry:
    %chosen_req=0;
    %chosen_len=0;
    if currentDev == DEV_ZKDM
    chosen_req = req_bytes_ZKDM;
    chosen_len    = req_len_ZKDM;
    chosen_expect_addr = expect_addr_ZKDM;
    chosen_expect_len  = expect_len_ZKDM;
    chosen_expect_crc  = expect_crc_kind_ZKDM;
    timeout_ms = timeout_ms_ZKDM;
    grant_ZKDM = true;
    grant_THERMO = false;
    elseif currentDev == DEV_THERMO
    chosen_req = req_bytes_THERMO;
    chosen_len = req_len_THERMO;
    chosen_expect_addr = expect_addr_THERMO;
    chosen_expect_len  = expect_len_THERMO;
    chosen_expect_crc  = expect_crc_kind_THERMO;
    timeout_ms = timeout_ms_THERMO;
    grant_ZKDM = false;
    grant_THERMO = true;
    end
    TX_Data = chosen_req;
    TX_Len = chosen_len;
    retry = 0; rxCount = 0;
  state BACKOFF
    entry:
    % prepare next cycle selection
    if currentDev==DEV_ZKDM
    % advance thermostat poll counter
    pollCounter = min(pollCounter+1, pollThermoEvery-1);
    end
  state WAIT_THRE
  state TX_PULSE
    entry:
    TX_Trigger = true;
  state WAIT_RX_SWITCH
  state DELIVER_OK_CLEAR
    entry:
    resp_ok_ZKDM = false;
    resp_ok_THERMO = false;
  state DELIVER_OK_PULSE
  state TX_CLEAR
    entry:
    TX_Trigger = false;
  state WAIT_RX [commented out]
    during:
    % append latest chunk
    if RX_Len > 0
    if (rxCount + RX_Len) <= length(rxBuf)
    rxBuf(rxCount+1 : rxCount+RX_Len) = RX_Data(1:RX_Len);
    rxCount = rxCount + RX_Len;
    else
    % overflow protection
    if currentDev==DEV_ZKDM
    err_ZKDM = ERR_OVERFLOW;
    else
    err_THERMO = ERR_OVERFLOW;
    end
    % consume and move on
    rxCount = 0;
    goto('BACKOFF');
    end
    end
  note: goes to VALIDATE
  state WAIT_RX2
    (junction 397) -> (junction 396) [order 1] : [[(rxCount + RX_Len) <= length(rxBuf)] && RX_Len > 0 ]
    WAIT_RX2 -> (junction 397) [order 1]
    (junction 396) -> (junction 398) : {rxBuf(rxCount+1 : rxCount+RX_Len) = RX_Data(1:RX_Len);
        | rxCount = rxCount + RX_Len;}
    (junction 397) -> WAIT_RX2 [order 4] : [RX_Len == 0]
    (junction 397) -> (junction 400) [order 2] : [(rxCount + RX_Len) > length(rxBuf)]
    (junction 398) -> WAIT_RX2
    (junction 400) -> (junction 409) [order 1] : [currentDev==DEV_ZKDM]
    (junction 400) -> (junction 406) [order 2] : {err_THERMO = ERR_OVERFLOW;}
    (junction 409) -> (junction 410) : {err_ZKDM = ERR_OVERFLOW;}
    (junction 410) -> (junction 406)
  state RETRY_OR_BACKOFF1
    RETRY_OR_BACKOFF1 -> (junction 271) : [(after(1,tick))]
        | {rxBuf = zeros(1, 127, 'uint8');
        | rxCount = 0;}
    (junction 271) -> (junction 272) [order 1] : [retry < maxRetry]
    (junction 271) -> (junction 273) [order 2]
    (junction 272) -> (junction 274) : {retry = retry + 1;}
    (junction 274) -> (junction 273) [order 2]
    (junction 273) -> (junction 275)
  state VALIDATE [commented out]
    entry:
    okAddr = addr_ok(rxBuf, rxCount, chosen_expect_addr);
    okLen  = len_ok(rxCount, chosen_expect_len);
    okCrc  = crc_ok(rxBuf, rxCount, chosen_expect_crc);
    if ~okAddr
    if currentDev==DEV_ZKDM
    err_ZKDM = ERR_BAD_ADDR;
    else
    err_THERMO = ERR_BAD_ADDR;
    end
    goto('RETRY_OR_BACKOFF');
    elseif ~okLen
    if currentDev==DEV_ZKDM
    err_ZKDM = ERR_BAD_LEN;
    else
    err_THERMO = ERR_BAD_LEN;
    end
    goto('RETRY_OR_BACKOFF');
    elseif ~okCrc
    if currentDev==DEV_ZKDM
    err_ZKDM = ERR_BAD_CRC;
    else
    err_THERMO = ERR_BAD_CRC;
    end
    goto('RETRY_OR_BACKOFF');
    else
    % success → deliver
    resp_data = rxBuf(1:rxCount);
    resp_len = rxCount;
    if currentDev==DEV_ZKDM
    resp_ok_ZKDM = true;
    else
    resp_ok_THERMO = true;
    end
    goto('DELIVER_OK_PULSE');
    end
  state DELIVER_ERROR
    entry:
    if currentDev==DEV_ZKDM
    resp_err_ZKDM = err_ZKDM;
    else
    resp_err_THERMO = err_THERMO;
    end
  note: goes to RETRY_OR_BACKOFF1
  note: goes to DELIVER_ERR
  state DELIVER_ERR
    entry:
    if currentDev==DEV_ZKDM
    err_ZKDM = ERR_TIMEOUT;
    else
    err_THERMO = ERR_TIMEOUT;
    end
  state RETRY_OR_BACKOFF [commented out]
    entry:
    if retry < maxRetry
    retry = retry + 1;
    % Re-transmit same chosen_req
    goto('WAIT_THRE');
    else
    % give up and move on
    goto('BACKOFF');
    end
  state WAIT_RX1 [commented out]
    (junction 318) -> (junction 144) [commented out] : [(rxCount + RX_Len) <= length(rxBuf)]
    (junction 148) -> (junction 318) [commented out] : [RX_Len > 0]
    (junction 148) -> (junction 327) [commented out] : [after(timeout_ms, msec)]
    (junction 144) -> (junction 139) [commented out] : {rxBuf(rxCount+1 : rxCount+RX_Len) = RX_Data(1:RX_Len);
        |  rxCount = rxCount + RX_Len;}
    (junction 318) -> (junction 141) [commented out]
    (junction 141) -> (junction 142) [commented out] : [currentDev==DEV_ZKDM]
    (junction 141) -> (junction 138) [commented out] : {err_THERMO = ERR_OVERFLOW;}
    (junction 142) -> (junction 143) [commented out] : {err_ZKDM = ERR_OVERFLOW;}
    (junction 143) -> (junction 138) [commented out]
    (junction 138) -> (junction 319) [commented out] : {rxCount = 0;}
    (junction 319) -> (junction 327) [commented out]
    (junction 139) -> (junction 319) [commented out]
  (default) -> INIT
  INIT -> IDLE : [(after(1,tick))]
  BACKOFF -> IDLE : [after(interGap_ms, msec)]
  IDLE -> IDLE [commented out] : [currentDev==DEV_NONE]
  (junction 397) -> (junction 256) [order 3] : [rxCount >= chosen_expect_len]
  IDLE -> LOAD_REQ [order 1] : [currentDev==DEV_ZKDM]
  IDLE -> LOAD_REQ [order 2] : [currentDev==DEV_THERMO]
  LOAD_REQ -> WAIT_THRE : [(after(1,tick))]
  DELIVER_ERROR -> BACKOFF
  DELIVER_OK_CLEAR -> BACKOFF
  (junction 274) -> WAIT_THRE [order 1]
  WAIT_THRE -> TX_PULSE [order 1] : [THRE==true && tx_switch]
  WAIT_RX_SWITCH -> WAIT_THRE [order 1] : [tx_switch]
  WAIT_THRE -> WAIT_RX_SWITCH [order 2] : [~tx_switch]
  (junction 235) -> RETRY_OR_BACKOFF1 [order 1]
  (junction 202) -> DELIVER_OK_PULSE
  TX_PULSE -> TX_CLEAR : [(after(1,tick))]
  WAIT_RX_SWITCH -> WAIT_RX2 [order 2] : [rx_switch]
  DELIVER_OK_PULSE -> DELIVER_OK_CLEAR : [(after(1,tick))]
  TX_CLEAR -> WAIT_RX2
  (junction 275) -> DELIVER_ERROR
  DELIVER_ERR -> RETRY_OR_BACKOFF1
  (junction 406) -> RETRY_OR_BACKOFF1
  WAIT_RX2 -> DELIVER_ERR [order 1] : [after(timeout_ms, msec)]
  data: buf function_input; count function_input; expect_addr function_input; ok function_output; count function_input; expect_len function_input; ok function_output; buf function_input; count function_input; expected_crc function_input; ok function_output; THRE input boolean size=1; RX_Data input uint8 size=[1 127]; RX_Len input uint8 size=1; req_valid_ZKDM input boolean size=1; req_valid_THERMO input boolean size=1; now input size=1; TX_Data output uint8 size=[1 127]; TX_Len output uint8 size=1; TX_Trigger output boolean size=1; grant_ZKDM output boolean size=1; resp_err_ZKDM output uint8 size=1; resp_ok_ZKDM output boolean size=1; resp_data output uint8 size=[1 127]; resp_err_THERMO output uint8 size=1; resp_len output uint8 size=1; grant_THERMO output boolean size=1; resp_ok_THERMO output boolean size=1; expect_addr_THERMO input uint8 size=1; expect_addr_ZKDM input uint8 size=1; expect_crc_kind_THERMO input uint8 size=1; expect_crc_kind_ZKDM input uint8 size=1; tx_switch input boolean size=1; rx_switch input boolean size=1; expect_len_THERMO input uint8 size=1; expect_len_ZKDM input uint8 size=1; req_bytes_THERMO input uint8 size=[1 127]; req_bytes_ZKDM input uint8 size=[1 127]; req_len_THERMO input uint8 size=1; req_len_ZKDM input uint8 size=1; interGap_ms local uint16 =5; maxRetry local uint8 =1; pollThermoEvery local uint8 =4; timeout_ms_THERMO local uint16 =80; timeout_ms_ZKDM local uint16 =20; chosen_expect_addr local uint8; chosen_expect_crc local uint8 size=1; chosen_expect_len local uint8 size=1; chosen_len local uint8 size=1; chosen_req local uint8 size=[1 127]; currentDev local uint8 size=1 =0; okAddr local boolean size=1; okCrc local boolean size=1; okLen local boolean size=1; pollCounter local uint8 size=1 =0; retry local uint8 size=1 =0; rxBuf local uint8 size=[1 127]; rxCount local uint8 size=1 =0; timeout_ms local uint16 size=1 =20; DEV_NONE constant uint8 =0; DEV_THERMO constant uint8 =2; DEV_ZKDM constant uint8 =1; ERR_BAD_ADDR constant uint8 =2; ERR_BAD_CRC constant uint8 =4; ERR_BAD_LEN constant uint8 =3; ERR_OVERFLOW constant uint8 =5; ERR_TIMEOUT constant uint8 =1; err_THERMO local uint8 size=1; err_ZKDM local uint8 size=1
  function ok = addr_ok(buf, count, expect_addr):
    | function ok = addr_ok(buf, count, expect_addr)
    |     if count < 3
    |         ok = false;
    |     else
    |         ok = (buf(3) == expect_addr);
    |     end
    | end
  function ok = len_ok(count, expect_len):
    | function ok = len_ok(count, expect_len)
    |     ok = (count == expect_len);
    | end
  function ok = crc_ok(buf, count, expected_crc):
    | function ok = crc_ok(buf, count, expected_crc)
    |     % kind: 0=BCC XOR, 1=CRC16-RTU (LSB first)
    |      bcc = uint8(0);
    |     for k=1:(count-1)
    |         bcc = bitxor(bcc, buf(k));
    |     end
    |     ok = (buf(count) == bcc);
    | end
